simulink model "MPC_control"  (R2018a)
settings: Solver=FixedStepAuto  StartTime=0  StopTime=Tend  FixedStep=0.001  RelTol=5e-3
model workspace (MAT data in the model file):
  A_mu = 10
  B_reff = 8.386
  Cz = 7766.25
  DCT_Param : struct (value not decoded)
  D_reff = 0.25826
  Downshift_Speeds = [9.5625 12.9375 16.3125 19.6875 23.0625 26.4375 29.8125 33.1875 36.5625 39.9375 43.3125 46.6875 ... (28 elements, 4x7)]
  Pedal_Positions = [0.1 0.4 0.5 0.9]
  SUS : struct (value not decoded)
  Upshift_Speeds = [12.9375 16.3125 19.6875 33 26.4375 29.8125 33.1875 52.5 39.9375 43.3125 46.6875 77.25 ... (28 elements, 4x7)]
  VEH : struct (value not decoded)
  V_o = 16.7
  V_xlow = 1
  WH : struct (value not decoded)
  a = 1.4
  alpha_max = 1.5
  alpha_min = -1.5
  b = 1.8
  c_zo = 209651
  epsilon = 0.1
  h = 0.134
  path : struct (value not decoded)
  pio = 220000
  q_Fcx = 0
  q_Fz2 = 15.4
  q_Fzy = 0
  q_reo = 0.9974
  q_sx1 = -0.007764
  q_sx10 = 0.2824
  q_sx11 = 5.349
  q_sx12 = 0
  q_sx13 = 0
  q_sx14 = 0
  q_sx2 = 1.1915
  q_sx3 = 0.013948
  q_sx4 = 4.912
  q_sx5 = 1.02
  q_sx6 = 22.83
  q_sx7 = 0.7104
  q_sx8 = -0.023393
  q_sx9 = 0.6581
  q_sy1 = 0.00702
  q_sy2 = 0
  q_sy3 = 0.001515
  q_sy4 = 8.514e-05
  q_sy5 = 0
  q_sy6 = 0
  q_sy7 = 0.9008
  q_sy8 = -0.4089
  q_v1 = 0.0007742
  q_v2 = 0.04667
  r_Bx1 = 12.531
  r_Bx2 = 9.532
  r_Bx3 = 0
  r_By1 = 10.615
  r_By2 = 7.705
  r_By3 = 3.433e-06
  r_By4 = 0
  r_Cx1 = 1.019
  r_Cy1 = 1.0585
  r_Ex1 = -0.4487
  r_Ex2 = -0.4726
  r_Ey1 = 0.3132
  r_Ey2 = 7.63e-06
  r_Hx1 = 0.0002374
  r_Hy1 = 0.011646
  r_Hy2 = 7.63e-06
  r_Vy1 = 0.05654
  r_Vy2 = 7.63e-06
  r_Vy3 = 0
  r_Vy4 = 99.9
  r_Vy5 = 2
  r_Vy6 = 15.814
  r_o = 0.3135
  vehWidth = 2
  w = 1
symbols that are objects in the model workspace (value not decoded): VEH
undefined symbols (not defined in the file): Cok_1, Cok_2, Cok_3, Cok_4, Cok_5, Cok_6, Cok_7, Cok_8, Cok_9, Cout_1, Cout_2, Cout_3, Cout_4, Cout_5, Cout_6, Cout_7, Cout_8, Cout_9, DiscIntNeverNeededParam, Dout_1, Dout_2, Dout_3, Dout_4, Dout_5, Dout_6, Dout_7, Dout_8, Dout_9, F_1, F_2, F_3, F_4, F_5, F_6, F_7, F_8, F_9, Gd_1, Gd_2, Gd_3, Gd_4, Gd_5, Gd_6, Gd_7, Gd_8, Gd_9, Gok_1, Gok_2, Gok_3, Gok_4, Gok_5, Gok_6, Gok_7, Gok_8, Gok_9, Gsys_2, Gsys_9, Hd_1, Hd_2, Hd_3 ... (+70)
libraries: robotalgslib x10, simulink x5, sim3dlib x2, autolibutils x1, vehdynlibviscommon x1
(part 4 of 5)

== system MPC_control/observer_of_plant/Subsystem_3/simulator_3/VH2P ==
  Velocities : Inport
  HeadingAngles : Inport  Port=2
  Initial position : Inport  Port=3
  Iintial Velocities : Inport  Port=4
  Iintial HeadingAngles : Inport  Port=5
  select_overlap : Inport  Port=6
  From Workspace1 : FromWorkspace  VariableName=Tsim  SampleTime=Ts
  Resettable Delay1 : Delay  DelayLength=1  InitialConditionSource=Input port  ExternalReset=Rising  SampleTime=Ts
      settings: InputPortMap=u0,r5,p4
  Resettable Delay2 : Delay  DelayLength=1  InitialConditionSource=Input port  ExternalReset=Rising  SampleTime=Ts
      settings: InputPortMap=u0,r5,p4
  Resettable Delay3 : Delay  DelayLength=1  InitialConditionSource=Input port  ExternalReset=Rising  SampleTime=Ts
      settings: InputPortMap=u0,r5,p4
  To Workspace : ToWorkspace  VariableName=Heading3  SampleTime=-1
  To Workspace1 : ToWorkspace  VariableName=Velocity3  SampleTime=-1
  To Workspace2 : ToWorkspace  VariableName=LastVelocity3  SampleTime=-1
  To Workspace3 : ToWorkspace  VariableName=Lastposition3  SampleTime=-1
  To Workspace4 : ToWorkspace  VariableName=LastHeading3  SampleTime=-1
  Unit Delay2 : UnitDelay  SampleTime=Ts
  YV2P : MATLAB Function  TreatAsAtomicUnit=on  SystemSampleTime=Ts
  Position : Outport
  wires:
  Velocities/1 -> Resettable Delay1/1, To Workspace1/1, YV2P/1(Velocity)
  Resettable Delay1/1 -> YV2P/2(LastVelocity), To Workspace2/1
  HeadingAngles/1 -> Resettable Delay2/1, To Workspace/1, YV2P/3(Heading)
  Resettable Delay2/1 -> YV2P/4(LastHeading), To Workspace4/1
  Initial position/1 -> Resettable Delay3/3
  Iintial Velocities/1 -> Resettable Delay1/3
  Iintial HeadingAngles/1 -> Resettable Delay2/3
  select_overlap/1 -> Resettable Delay3/2, Resettable Delay2/2, Resettable Delay1/2
  From Workspace1/1 -> YV2P/5(Tsim), Unit Delay2/1
  Unit Delay2/1 -> YV2P/6(LastTsim)
  Resettable Delay3/1 -> YV2P/7(Lastpostion), To Workspace3/1
  YV2P/1(Position) -> Resettable Delay3/1, Position/1

== system MPC_control/observer_of_plant/Subsystem_3/simulator_3/YV_update ==
  XY_sim : Inport
  Velocity_sim : Inport  Port=2
  Heading_sim : Inport  Port=3
  Constant : Constant  Value=Ts  SampleTime=Ts
  Discrete-Time Integrator : DiscreteIntegrator  Commented=on  SampleTime=Ts  ICPrevOutput=DiscIntNeverNeededParam  ICPrevScaledInput=DiscIntNeverNeededParam
  From Workspace1 : FromWorkspace  VariableName=Tsim  SampleTime=Ts
  From Workspace3 : FromWorkspace  VariableName=XYplot_ref  SampleTime=Ts
  Gain : Gain  Commented=on  Gain=[eye(2), zeros(2,10)]  Multiplication=Matrix(K*u) (u vector)
  Mux : Mux  Commented=on  Inputs=2
  Pure Pursuit : robotalgslib/Pure Pursuit  Commented=on  DesiredLinearVelocity=0.1  MaxAngularVelocity=1.0  LookaheadDistance=2.5  TargetDirPort=off  SimulateUsing=Code generation
      settings: SourceProductName=Robotics System Toolbox  SourceProductBaseCode=RO
  Transpose : Math  Commented=on  Operator=transpose  SaturateOnIntegerOverflow=on
  YV_update : MATLAB Function  TreatAsAtomicUnit=on  SystemSampleTime=Ts
  Velocity_updated : Outport
  Heading_updated : Outport  Port=2
  wires:
  YV_update/1(Velocity_updated) -> Velocity_updated/1
  From Workspace1/1 -> YV_update/6(Tsim)
  Velocity_sim/1 -> YV_update/3(Velocity_sim)
  Constant/1 -> YV_update/5(Ts)
  Pure Pursuit/2 -> Discrete-Time Integrator/1
  Heading_sim/1 -> Mux/2, YV_update/4(Heading_sim)
  Mux/1 -> Pure Pursuit/1
  From Workspace3/1 -> Gain/1, YV_update/1(XYplot_ref)
  XY_sim/1 -> Mux/1, YV_update/2(XYplot_sim)
  Gain/1 -> Transpose/1
  Transpose/1 -> Pure Pursuit/2
  YV_update/2(Heading_updated) -> Heading_updated/1

== system MPC_control/observer_of_plant/Subsystem_4/simulator_4/MPC_of_simulator_4 ==
  Velocity_updated : Inport  SampleTime=Ts  LockScale=on
  Heading_updated : Inport  Port=2  SampleTime=Ts  LockScale=on
  Xhat : Inport  Port=3
  U(k-1) : Inport  Port=4  SampleTime=Ts  LockScale=on
  select_MPC : Inport  Port=5  SampleTime=Ts  LockScale=on
  select_overlap : Inport  Port=6  SampleTime=Ts  LockScale=on
  Clock : Clock
  Constant1 : Constant  Value=M  VectorParams1D=off  SampleTime=-1
  Constant2 : Constant  Value=Np  SampleTime=-1
  Constant3 : Constant  Value=JE_4  VectorParams1D=off  SampleTime=-1
  Constant4 : Constant  Value=Qc_4  VectorParams1D=off  SampleTime=-1
  Constant5 : Constant  Value=phi_4  VectorParams1D=off  SampleTime=-1
  F_Middle : Gain  Gain=F_4  Multiplication=Matrix(K*u) (u vector)
  From Workspace6 : FromWorkspace  VariableName=Rs  SampleTime=Ts
  HQP : MATLAB Function  TreatAsAtomicUnit=on  SystemSampleTime=Ts
  Resettable Delay2 : Delay  DelayLength=1  InitialConditionSource=Input port  ExternalReset=Rising  SampleTime=Ts
      settings: InputPortMap=u0,r5,p4
  r(k+1) : Outport
  U : Outport  Port=2
  wires:
  HQP/2(U) -> Resettable Delay2/1, U/1
  Xhat/1 -> F_Middle/1
  Constant4/1 -> HQP/4(Qc)
  Constant5/1 -> HQP/2(phi)
  Constant3/1 -> HQP/1(JE)
  Constant2/1 -> HQP/6(Np)
  Constant1/1 -> HQP/5(M)
  Clock/1 -> HQP/10(Tsim)
  F_Middle/1 -> HQP/3(Fxh)
  From Workspace6/1 -> HQP/9(Rs)
  Heading_updated/1 -> HQP/7(Heading_updated)
  Velocity_updated/1 -> HQP/8(Velocity_updated)
  HQP/1(r) -> r(k+1)/1
  select_MPC/1 -> HQP/11(select_MPC)
  Resettable Delay2/1 -> HQP/12(U_delay)
  select_overlap/1 -> HQP/13(select_overlap), Resettable Delay2/2
  U(k-1)/1 -> Resettable Delay2/3

== system MPC_control/observer_of_plant/Subsystem_4/simulator_4/VH2P ==
  Velocities : Inport
  HeadingAngles : Inport  Port=2
  Initial position : Inport  Port=3
  Iintial Velocities : Inport  Port=4
  Iintial HeadingAngles : Inport  Port=5
  select_overlap : Inport  Port=6
  From Workspace1 : FromWorkspace  VariableName=Tsim  SampleTime=Ts
  Resettable Delay1 : Delay  DelayLength=1  InitialConditionSource=Input port  ExternalReset=Rising  SampleTime=Ts
      settings: InputPortMap=u0,r5,p4
  Resettable Delay2 : Delay  DelayLength=1  InitialConditionSource=Input port  ExternalReset=Rising  SampleTime=Ts
      settings: InputPortMap=u0,r5,p4
  Resettable Delay3 : Delay  DelayLength=1  InitialConditionSource=Input port  ExternalReset=Rising  SampleTime=Ts
      settings: InputPortMap=u0,r5,p4
  Unit Delay2 : UnitDelay  SampleTime=Ts
  YV2P : MATLAB Function  TreatAsAtomicUnit=on  SystemSampleTime=Ts
  Position : Outport
  wires:
  YV2P/1(Position) -> Resettable Delay3/1, Position/1
  Velocities/1 -> Resettable Delay1/1, YV2P/1(Velocity)
  Resettable Delay1/1 -> YV2P/2(LastVelocity)
  HeadingAngles/1 -> Resettable Delay2/1, YV2P/3(Heading)
  Resettable Delay2/1 -> YV2P/4(LastHeading)
  Resettable Delay3/1 -> YV2P/7(Lastpostion)
  Initial position/1 -> Resettable Delay3/3
  Iintial Velocities/1 -> Resettable Delay1/3
  Iintial HeadingAngles/1 -> Resettable Delay2/3
  select_overlap/1 -> Resettable Delay3/2, Resettable Delay2/2, Resettable Delay1/2
  From Workspace1/1 -> YV2P/5(Tsim), Unit Delay2/1
  Unit Delay2/1 -> YV2P/6(LastTsim)

== system MPC_control/observer_of_plant/Subsystem_4/simulator_4/YV_update ==
  XY_sim : Inport
  Velocity_sim : Inport  Port=2
  Heading_sim : Inport  Port=3
  Constant : Constant  Value=Ts  SampleTime=Ts
  Discrete-Time Integrator : DiscreteIntegrator  Commented=on  SampleTime=Ts  ICPrevOutput=DiscIntNeverNeededParam  ICPrevScaledInput=DiscIntNeverNeededParam
  From Workspace1 : FromWorkspace  VariableName=Tsim  SampleTime=Ts
  From Workspace3 : FromWorkspace  VariableName=XYplot_ref  SampleTime=Ts
  Gain : Gain  Commented=on  Gain=[eye(2), zeros(2,10)]  Multiplication=Matrix(K*u) (u vector)
  Mux : Mux  Commented=on  Inputs=2
  Pure Pursuit : robotalgslib/Pure Pursuit  Commented=on  DesiredLinearVelocity=0.1  MaxAngularVelocity=1.0  LookaheadDistance=2.5  TargetDirPort=off  SimulateUsing=Code generation
      settings: SourceProductName=Robotics System Toolbox  SourceProductBaseCode=RO
  Transpose : Math  Commented=on  Operator=transpose  SaturateOnIntegerOverflow=on
  YV_update : MATLAB Function  TreatAsAtomicUnit=on  SystemSampleTime=Ts
  Velocity_updated : Outport
  Heading_updated : Outport  Port=2
  wires:
  From Workspace1/1 -> YV_update/6(Tsim)
  Velocity_sim/1 -> YV_update/3(Velocity_sim)
  Constant/1 -> YV_update/5(Ts)
  Pure Pursuit/2 -> Discrete-Time Integrator/1
  Heading_sim/1 -> Mux/2, YV_update/4(Heading_sim)
  From Workspace3/1 -> Gain/1, YV_update/1(XYplot_ref)
  Mux/1 -> Pure Pursuit/1
  YV_update/1(Velocity_updated) -> Velocity_updated/1
  Transpose/1 -> Pure Pursuit/2
  Gain/1 -> Transpose/1
  XY_sim/1 -> Mux/1, YV_update/2(XYplot_sim)
  YV_update/2(Heading_updated) -> Heading_updated/1

== system MPC_control/observer_of_plant/Subsystem_5/simulator_5/MPC_of_simulator_5 ==
  Velocity_updated : Inport  SampleTime=Ts  LockScale=on
  Heading_updated : Inport  Port=2  SampleTime=Ts  LockScale=on
  Xhat : Inport  Port=3
  U(k-1) : Inport  Port=4  SampleTime=Ts  LockScale=on
  select_MPC : Inport  Port=5  SampleTime=Ts  LockScale=on
  select_overlap : Inport  Port=6  SampleTime=Ts  LockScale=on
  Clock : Clock
  Constant1 : Constant  Value=M  VectorParams1D=off  SampleTime=-1
  Constant2 : Constant  Value=Np  SampleTime=-1
  Constant3 : Constant  Value=JE_5  VectorParams1D=off  SampleTime=-1
  Constant4 : Constant  Value=Qc_5  VectorParams1D=off  SampleTime=-1
  Constant5 : Constant  Value=phi_5  VectorParams1D=off  SampleTime=-1
  F_Middle : Gain  Gain=F_5  Multiplication=Matrix(K*u) (u vector)
  From Workspace6 : FromWorkspace  VariableName=Rs  SampleTime=Ts
  HQP : MATLAB Function  TreatAsAtomicUnit=on  SystemSampleTime=Ts
  Resettable Delay2 : Delay  DelayLength=1  InitialConditionSource=Input port  ExternalReset=Rising  SampleTime=Ts
      settings: InputPortMap=u0,r5,p4
  r(k+1) : Outport
  U : Outport  Port=2
  wires:
  HQP/2(U) -> Resettable Delay2/1, U/1
  Xhat/1 -> F_Middle/1
  Constant4/1 -> HQP/4(Qc)
  Constant5/1 -> HQP/2(phi)
  Constant3/1 -> HQP/1(JE)
  Constant2/1 -> HQP/6(Np)
  Constant1/1 -> HQP/5(M)
  Clock/1 -> HQP/10(Tsim)
  F_Middle/1 -> HQP/3(Fxh)
  From Workspace6/1 -> HQP/9(Rs)
  Heading_updated/1 -> HQP/7(Heading_updated)
  Velocity_updated/1 -> HQP/8(Velocity_updated)
  HQP/1(r) -> r(k+1)/1
  select_MPC/1 -> HQP/11(select_MPC)
  Resettable Delay2/1 -> HQP/12(U_delay)
  select_overlap/1 -> Resettable Delay2/2
  U(k-1)/1 -> Resettable Delay2/3

== system MPC_control/observer_of_plant/Subsystem_5/simulator_5/VH2P ==
  Velocities : Inport
  HeadingAngles : Inport  Port=2
  Initial position : Inport  Port=3
  Iintial Velocities : Inport  Port=4
  Iintial HeadingAngles : Inport  Port=5
  select_overlap : Inport  Port=6
  From Workspace1 : FromWorkspace  VariableName=Tsim  SampleTime=Ts
  Resettable Delay1 : Delay  DelayLength=1  InitialConditionSource=Input port  ExternalReset=Rising  SampleTime=Ts
      settings: InputPortMap=u0,r5,p4
  Resettable Delay2 : Delay  DelayLength=1  InitialConditionSource=Input port  ExternalReset=Rising  SampleTime=Ts
      settings: InputPortMap=u0,r5,p4
  Resettable Delay3 : Delay  DelayLength=1  InitialConditionSource=Input port  ExternalReset=Rising  SampleTime=Ts
      settings: InputPortMap=u0,r5,p4
  Unit Delay2 : UnitDelay  SampleTime=Ts
  YV2P : MATLAB Function  TreatAsAtomicUnit=on  SystemSampleTime=Ts
  Position : Outport
  wires:
  YV2P/1(Position) -> Resettable Delay3/1, Position/1
  Velocities/1 -> Resettable Delay1/1, YV2P/1(Velocity)
  Resettable Delay1/1 -> YV2P/2(LastVelocity)
  HeadingAngles/1 -> Resettable Delay2/1, YV2P/3(Heading)
  Resettable Delay2/1 -> YV2P/4(LastHeading)
  Resettable Delay3/1 -> YV2P/7(Lastpostion)
  Initial position/1 -> Resettable Delay3/3
  Iintial Velocities/1 -> Resettable Delay1/3
  Iintial HeadingAngles/1 -> Resettable Delay2/3
  select_overlap/1 -> Resettable Delay3/2, Resettable Delay2/2, Resettable Delay1/2
  From Workspace1/1 -> YV2P/5(Tsim), Unit Delay2/1
  Unit Delay2/1 -> YV2P/6(LastTsim)

== system MPC_control/observer_of_plant/Subsystem_5/simulator_5/YV_update ==
  XY_sim : Inport
  Velocity_sim : Inport  Port=2
  Heading_sim : Inport  Port=3
  Constant : Constant  Value=Ts  SampleTime=Ts
  Discrete-Time Integrator : DiscreteIntegrator  Commented=on  SampleTime=Ts  ICPrevOutput=DiscIntNeverNeededParam  ICPrevScaledInput=DiscIntNeverNeededParam
  From Workspace1 : FromWorkspace  VariableName=Tsim  SampleTime=Ts
  From Workspace3 : FromWorkspace  VariableName=XYplot_ref  SampleTime=Ts
  Gain : Gain  Commented=on  Gain=[eye(2), zeros(2,10)]  Multiplication=Matrix(K*u) (u vector)
  Mux : Mux  Commented=on  Inputs=2
  Pure Pursuit : robotalgslib/Pure Pursuit  Commented=on  DesiredLinearVelocity=0.1  MaxAngularVelocity=1.0  LookaheadDistance=2.5  TargetDirPort=off  SimulateUsing=Code generation
      settings: SourceProductName=Robotics System Toolbox  SourceProductBaseCode=RO
  Transpose : Math  Commented=on  Operator=transpose  SaturateOnIntegerOverflow=on
  YV_update : MATLAB Function  TreatAsAtomicUnit=on  SystemSampleTime=Ts
  Velocity_updated : Outport
  Heading_updated : Outport  Port=2
  wires:
  YV_update/1(Velocity_updated) -> Velocity_updated/1
  From Workspace1/1 -> YV_update/6(Tsim)
  Velocity_sim/1 -> YV_update/3(Velocity_sim)
  Constant/1 -> YV_update/5(Ts)
  Pure Pursuit/2 -> Discrete-Time Integrator/1
  Heading_sim/1 -> Mux/2, YV_update/4(Heading_sim)
  Mux/1 -> Pure Pursuit/1
  From Workspace3/1 -> Gain/1, YV_update/1(XYplot_ref)
  XY_sim/1 -> Mux/1, YV_update/2(XYplot_sim)
  Gain/1 -> Transpose/1
  Transpose/1 -> Pure Pursuit/2
  YV_update/2(Heading_updated) -> Heading_updated/1

== system MPC_control/observer_of_plant/Subsystem_6/simulator_6/MPC_of_simulator_6 ==
  Velocity_updated : Inport  SampleTime=Ts  LockScale=on
  Heading_updated : Inport  Port=2  SampleTime=Ts  LockScale=on
  Xhat : Inport  Port=3
  U(k-1) : Inport  Port=4  SampleTime=Ts  LockScale=on
  select_MPC : Inport  Port=5  SampleTime=Ts  LockScale=on
  select_overlap : Inport  Port=6  SampleTime=Ts  LockScale=on
  Clock : Clock
  Constant1 : Constant  Value=M  VectorParams1D=off  SampleTime=-1
  Constant2 : Constant  Value=Np  SampleTime=-1
  Constant3 : Constant  Value=JE_6  VectorParams1D=off  SampleTime=-1
  Constant4 : Constant  Value=Qc_6  VectorParams1D=off  SampleTime=-1
  Constant5 : Constant  Value=phi_6  VectorParams1D=off  SampleTime=-1
  F_Middle : Gain  Gain=F_6  Multiplication=Matrix(K*u) (u vector)
  From Workspace6 : FromWorkspace  VariableName=Rs  SampleTime=Ts
  HQP : MATLAB Function  TreatAsAtomicUnit=on  SystemSampleTime=Ts
  Resettable Delay2 : Delay  DelayLength=1  InitialConditionSource=Input port  ExternalReset=Rising  SampleTime=Ts
      settings: InputPortMap=u0,r5,p4
  r(k+1) : Outport
  U : Outport  Port=2
  wires:
  HQP/2(U) -> Resettable Delay2/1, U/1
  Xhat/1 -> F_Middle/1
  Constant4/1 -> HQP/4(Qc)
  Constant5/1 -> HQP/2(phi)
  Constant3/1 -> HQP/1(JE)
  Constant2/1 -> HQP/6(Np)
  Constant1/1 -> HQP/5(M)
  Clock/1 -> HQP/10(Tsim)
  F_Middle/1 -> HQP/3(Fxh)
  From Workspace6/1 -> HQP/9(Rs)
  Heading_updated/1 -> HQP/7(Heading_updated)
  Velocity_updated/1 -> HQP/8(Velocity_updated)
  HQP/1(r) -> r(k+1)/1
  select_MPC/1 -> HQP/11(select_MPC)
  Resettable Delay2/1 -> HQP/12(U_delay)
  select_overlap/1 -> Resettable Delay2/2
  U(k-1)/1 -> Resettable Delay2/3

== system MPC_control/observer_of_plant/Subsystem_6/simulator_6/VH2P ==
  Velocities : Inport
  HeadingAngles : Inport  Port=2
  Initial position : Inport  Port=3
  Iintial Velocities : Inport  Port=4
  Iintial HeadingAngles : Inport  Port=5
  select_overlap : Inport  Port=6
  From Workspace1 : FromWorkspace  VariableName=Tsim  SampleTime=Ts
  Resettable Delay1 : Delay  DelayLength=1  InitialConditionSource=Input port  ExternalReset=Rising  SampleTime=Ts
      settings: InputPortMap=u0,r5,p4
  Resettable Delay2 : Delay  DelayLength=1  InitialConditionSource=Input port  ExternalReset=Rising  SampleTime=Ts
      settings: InputPortMap=u0,r5,p4
  Resettable Delay3 : Delay  DelayLength=1  InitialConditionSource=Input port  ExternalReset=Rising  SampleTime=Ts
      settings: InputPortMap=u0,r5,p4
  Unit Delay2 : UnitDelay  SampleTime=Ts
  YV2P : MATLAB Function  TreatAsAtomicUnit=on  SystemSampleTime=Ts
  Position : Outport
  wires:
  YV2P/1(Position) -> Resettable Delay3/1, Position/1
  Velocities/1 -> Resettable Delay1/1, YV2P/1(Velocity)
  Resettable Delay1/1 -> YV2P/2(LastVelocity)
  HeadingAngles/1 -> Resettable Delay2/1, YV2P/3(Heading)
  Resettable Delay2/1 -> YV2P/4(LastHeading)
  Resettable Delay3/1 -> YV2P/7(Lastpostion)
  Initial position/1 -> Resettable Delay3/3
  Iintial Velocities/1 -> Resettable Delay1/3
  Iintial HeadingAngles/1 -> Resettable Delay2/3
  select_overlap/1 -> Resettable Delay3/2, Resettable Delay2/2, Resettable Delay1/2
  From Workspace1/1 -> YV2P/5(Tsim), Unit Delay2/1
  Unit Delay2/1 -> YV2P/6(LastTsim)

== system MPC_control/observer_of_plant/Subsystem_6/simulator_6/YV_update ==
  XY_sim : Inport
  Velocity_sim : Inport  Port=2
  Heading_sim : Inport  Port=3
  Constant : Constant  Value=Ts  SampleTime=Ts
  Discrete-Time Integrator : DiscreteIntegrator  Commented=on  SampleTime=Ts  ICPrevOutput=DiscIntNeverNeededParam  ICPrevScaledInput=DiscIntNeverNeededParam
  From Workspace1 : FromWorkspace  VariableName=Tsim  SampleTime=Ts
  From Workspace3 : FromWorkspace  VariableName=XYplot_ref  SampleTime=Ts
  Gain : Gain  Commented=on  Gain=[eye(2), zeros(2,10)]  Multiplication=Matrix(K*u) (u vector)
  Mux : Mux  Commented=on  Inputs=2
  Pure Pursuit : robotalgslib/Pure Pursuit  Commented=on  DesiredLinearVelocity=0.1  MaxAngularVelocity=1.0  LookaheadDistance=2.5  TargetDirPort=off  SimulateUsing=Code generation
      settings: SourceProductName=Robotics System Toolbox  SourceProductBaseCode=RO
  Transpose : Math  Commented=on  Operator=transpose  SaturateOnIntegerOverflow=on
  YV_update : MATLAB Function  TreatAsAtomicUnit=on  SystemSampleTime=Ts
  Velocity_updated : Outport
  Heading_updated : Outport  Port=2
  wires:
  YV_update/1(Velocity_updated) -> Velocity_updated/1
  From Workspace1/1 -> YV_update/6(Tsim)
  Velocity_sim/1 -> YV_update/3(Velocity_sim)
  Constant/1 -> YV_update/5(Ts)
  Pure Pursuit/2 -> Discrete-Time Integrator/1
  Heading_sim/1 -> Mux/2, YV_update/4(Heading_sim)
  Mux/1 -> Pure Pursuit/1
  From Workspace3/1 -> Gain/1, YV_update/1(XYplot_ref)
  XY_sim/1 -> Mux/1, YV_update/2(XYplot_sim)
  Gain/1 -> Transpose/1
  Transpose/1 -> Pure Pursuit/2
  YV_update/2(Heading_updated) -> Heading_updated/1

== system MPC_control/observer_of_plant/Subsystem_7/simulator_7/MPC_of_simulator_7 ==
  Velocity_updated : Inport  SampleTime=Ts  LockScale=on
  Heading_updated : Inport  Port=2  SampleTime=Ts  LockScale=on
  Xhat : Inport  Port=3
  U(k-1) : Inport  Port=4  SampleTime=Ts  LockScale=on
  select_MPC : Inport  Port=5  SampleTime=Ts  LockScale=on
  select_overlap : Inport  Port=6  SampleTime=Ts  LockScale=on
  Clock : Clock
  Constant1 : Constant  Value=M  VectorParams1D=off  SampleTime=-1
  Constant2 : Constant  Value=Np  SampleTime=-1
  Constant3 : Constant  Value=JE_7  VectorParams1D=off  SampleTime=-1
  Constant4 : Constant  Value=Qc_7  VectorParams1D=off  SampleTime=-1
  Constant5 : Constant  Value=phi_7  VectorParams1D=off  SampleTime=-1
  F_Middle : Gain  Gain=F_7  Multiplication=Matrix(K*u) (u vector)
  From Workspace6 : FromWorkspace  VariableName=Rs  SampleTime=Ts
  HQP : MATLAB Function  TreatAsAtomicUnit=on  SystemSampleTime=Ts
  Resettable Delay2 : Delay  DelayLength=1  InitialConditionSource=Input port  ExternalReset=Rising  SampleTime=Ts
      settings: InputPortMap=u0,r5,p4
  r(k+1) : Outport
  U : Outport  Port=2
  wires:
  HQP/2(U) -> Resettable Delay2/1, U/1
  Xhat/1 -> F_Middle/1
  Constant4/1 -> HQP/4(Qc)
  Constant5/1 -> HQP/2(phi)
  Constant3/1 -> HQP/1(JE)
  Constant2/1 -> HQP/6(Np)
  Constant1/1 -> HQP/5(M)
  Clock/1 -> HQP/10(Tsim)
  F_Middle/1 -> HQP/3(Fxh)
  From Workspace6/1 -> HQP/9(Rs)
  Heading_updated/1 -> HQP/7(Heading_updated)
  Velocity_updated/1 -> HQP/8(Velocity_updated)
  HQP/1(r) -> r(k+1)/1
  select_MPC/1 -> HQP/11(select_MPC)
  Resettable Delay2/1 -> HQP/12(U_delay)
  select_overlap/1 -> Resettable Delay2/2
  U(k-1)/1 -> Resettable Delay2/3

== system MPC_control/observer_of_plant/Subsystem_7/simulator_7/VH2P ==
  Velocities : Inport
  HeadingAngles : Inport  Port=2
  Initial position : Inport  Port=3
  Iintial Velocities : Inport  Port=4
  Iintial HeadingAngles : Inport  Port=5
  select_overlap : Inport  Port=6
  From Workspace1 : FromWorkspace  VariableName=Tsim  SampleTime=Ts
  Resettable Delay1 : Delay  DelayLength=1  InitialConditionSource=Input port  ExternalReset=Rising  SampleTime=Ts
      settings: InputPortMap=u0,r5,p4
  Resettable Delay2 : Delay  DelayLength=1  InitialConditionSource=Input port  ExternalReset=Rising  SampleTime=Ts
      settings: InputPortMap=u0,r5,p4
  Resettable Delay3 : Delay  DelayLength=1  InitialConditionSource=Input port  ExternalReset=Rising  SampleTime=Ts
      settings: InputPortMap=u0,r5,p4
  Unit Delay2 : UnitDelay  SampleTime=Ts
  YV2P : MATLAB Function  TreatAsAtomicUnit=on  SystemSampleTime=Ts
  Position : Outport
  wires:
  YV2P/1(Position) -> Resettable Delay3/1, Position/1
  Resettable Delay2/1 -> YV2P/4(LastHeading)
  Resettable Delay3/1 -> YV2P/7(Lastpostion)
  Initial position/1 -> Resettable Delay3/3
  Iintial Velocities/1 -> Resettable Delay1/3
  Iintial HeadingAngles/1 -> Resettable Delay2/3
  select_overlap/1 -> Resettable Delay3/2, Resettable Delay2/2, Resettable Delay1/2
  From Workspace1/1 -> YV2P/5(Tsim), Unit Delay2/1
  Unit Delay2/1 -> YV2P/6(LastTsim)
  Resettable Delay1/1 -> YV2P/2(LastVelocity)
  HeadingAngles/1 -> Resettable Delay2/1, YV2P/3(Heading)
  Velocities/1 -> Resettable Delay1/1, YV2P/1(Velocity)

== system MPC_control/observer_of_plant/Subsystem_7/simulator_7/YV_update ==
  XY_sim : Inport
  Velocity_sim : Inport  Port=2
  Heading_sim : Inport  Port=3
  Constant : Constant  Value=Ts  SampleTime=Ts
  Discrete-Time Integrator : DiscreteIntegrator  Commented=on  SampleTime=Ts  ICPrevOutput=DiscIntNeverNeededParam  ICPrevScaledInput=DiscIntNeverNeededParam
  From Workspace1 : FromWorkspace  VariableName=Tsim  SampleTime=Ts
  From Workspace3 : FromWorkspace  VariableName=XYplot_ref  SampleTime=Ts
  Gain : Gain  Commented=on  Gain=[eye(2), zeros(2,10)]  Multiplication=Matrix(K*u) (u vector)
  Mux : Mux  Commented=on  Inputs=2
  Pure Pursuit : robotalgslib/Pure Pursuit  Commented=on  DesiredLinearVelocity=0.1  MaxAngularVelocity=1.0  LookaheadDistance=2.5  TargetDirPort=off  SimulateUsing=Code generation
      settings: SourceProductName=Robotics System Toolbox  SourceProductBaseCode=RO
  Transpose : Math  Commented=on  Operator=transpose  SaturateOnIntegerOverflow=on
  YV_update : MATLAB Function  TreatAsAtomicUnit=on  SystemSampleTime=Ts
  Velocity_updated : Outport
  Heading_updated : Outport  Port=2
  wires:
  From Workspace1/1 -> YV_update/6(Tsim)
  Velocity_sim/1 -> YV_update/3(Velocity_sim)
  Constant/1 -> YV_update/5(Ts)
  Pure Pursuit/2 -> Discrete-Time Integrator/1
  Heading_sim/1 -> Mux/2, YV_update/4(Heading_sim)
  From Workspace3/1 -> Gain/1, YV_update/1(XYplot_ref)
  YV_update/1(Velocity_updated) -> Velocity_updated/1
  Mux/1 -> Pure Pursuit/1
  Transpose/1 -> Pure Pursuit/2
  Gain/1 -> Transpose/1
  XY_sim/1 -> Mux/1, YV_update/2(XYplot_sim)
  YV_update/2(Heading_updated) -> Heading_updated/1

== system MPC_control/observer_of_plant/Subsystem_8/simulator_8/MPC_of_simulator_8 ==
  Velocity_updated : Inport  SampleTime=Ts  LockScale=on
  Heading_updated : Inport  Port=2  SampleTime=Ts  LockScale=on
  Xhat : Inport  Port=3
  U(k-1) : Inport  Port=4  SampleTime=Ts  LockScale=on
  select_MPC : Inport  Port=5  SampleTime=Ts  LockScale=on
  select_overlap : Inport  Port=6  SampleTime=Ts  LockScale=on
  Clock : Clock
  Constant1 : Constant  Value=M  VectorParams1D=off  SampleTime=-1
  Constant2 : Constant  Value=Np  SampleTime=-1
  Constant3 : Constant  Value=JE_8  VectorParams1D=off  SampleTime=-1
  Constant4 : Constant  Value=Qc_8  VectorParams1D=off  SampleTime=-1
  Constant5 : Constant  Value=phi_8  VectorParams1D=off  SampleTime=-1
  F_Middle1 : Gain  Gain=F_8  Multiplication=Matrix(K*u) (u vector)
  From Workspace6 : FromWorkspace  VariableName=Rs  SampleTime=Ts
  HQP : MATLAB Function  TreatAsAtomicUnit=on  SystemSampleTime=Ts
  Resettable Delay2 : Delay  DelayLength=1  InitialConditionSource=Input port  ExternalReset=Rising  SampleTime=Ts
      settings: InputPortMap=u0,r5,p4
  r(k+1) : Outport
  U : Outport  Port=2
  wires:
  HQP/2(U) -> Resettable Delay2/1, U/1
  Constant4/1 -> HQP/4(Qc)
  Constant5/1 -> HQP/2(phi)
  Constant3/1 -> HQP/1(JE)
  Constant2/1 -> HQP/6(Np)
  Constant1/1 -> HQP/5(M)
  Clock/1 -> HQP/10(Tsim)
  F_Middle1/1 -> HQP/3(Fxh)
  From Workspace6/1 -> HQP/9(Rs)
  Heading_updated/1 -> HQP/7(Heading_updated)
  Velocity_updated/1 -> HQP/8(Velocity_updated)
  HQP/1(r) -> r(k+1)/1
  select_MPC/1 -> HQP/11(select_MPC)
  Resettable Delay2/1 -> HQP/12(U_delay)
  select_overlap/1 -> Resettable Delay2/2
  U(k-1)/1 -> Resettable Delay2/3
  Xhat/1 -> F_Middle1/1

== system MPC_control/observer_of_plant/Subsystem_8/simulator_8/VH2P ==
  Velocities : Inport
  HeadingAngles : Inport  Port=2
  Initial position : Inport  Port=3
  Iintial Velocities : Inport  Port=4
  Iintial HeadingAngles : Inport  Port=5
  select_overlap : Inport  Port=6
  From Workspace1 : FromWorkspace  VariableName=Tsim  SampleTime=Ts
  Resettable Delay1 : Delay  DelayLength=1  InitialConditionSource=Input port  ExternalReset=Rising  SampleTime=Ts
      settings: InputPortMap=u0,r5,p4
  Resettable Delay2 : Delay  DelayLength=1  InitialConditionSource=Input port  ExternalReset=Rising  SampleTime=Ts
      settings: InputPortMap=u0,r5,p4
  Resettable Delay3 : Delay  DelayLength=1  InitialConditionSource=Input port  ExternalReset=Rising  SampleTime=Ts
      settings: InputPortMap=u0,r5,p4
  To Workspace : ToWorkspace  VariableName=Heading8  SampleTime=-1
  To Workspace1 : ToWorkspace  VariableName=Velocity8  SampleTime=-1
  To Workspace2 : ToWorkspace  VariableName=LastVelocity8  SampleTime=-1
  To Workspace3 : ToWorkspace  VariableName=Lastposition8  SampleTime=-1
  To Workspace4 : ToWorkspace  VariableName=LastHeading8  SampleTime=-1
  Unit Delay2 : UnitDelay  SampleTime=Ts
  YV2P : MATLAB Function  TreatAsAtomicUnit=on  SystemSampleTime=Ts
  Position : Outport
  wires:
  YV2P/1(Position) -> Resettable Delay3/1, Position/1
  Velocities/1 -> Resettable Delay1/1, To Workspace1/1, YV2P/1(Velocity)
  Resettable Delay1/1 -> To Workspace2/1, YV2P/2(LastVelocity)
  HeadingAngles/1 -> Resettable Delay2/1, To Workspace/1, YV2P/3(Heading)
  Resettable Delay2/1 -> To Workspace4/1, YV2P/4(LastHeading)
  Resettable Delay3/1 -> To Workspace3/1, YV2P/7(Lastpostion)
  Initial position/1 -> Resettable Delay3/3
  Iintial Velocities/1 -> Resettable Delay1/3
  Iintial HeadingAngles/1 -> Resettable Delay2/3
  select_overlap/1 -> Resettable Delay3/2, Resettable Delay2/2, Resettable Delay1/2
  From Workspace1/1 -> YV2P/5(Tsim), Unit Delay2/1
  Unit Delay2/1 -> YV2P/6(LastTsim)

== system MPC_control/observer_of_plant/Subsystem_8/simulator_8/YV_update ==
  XY_sim : Inport
  Velocity_sim : Inport  Port=2
  Heading_sim : Inport  Port=3
  Constant : Constant  Value=Ts  SampleTime=Ts
  Discrete-Time Integrator : DiscreteIntegrator  Commented=on  SampleTime=Ts  ICPrevOutput=DiscIntNeverNeededParam  ICPrevScaledInput=DiscIntNeverNeededParam
  From Workspace1 : FromWorkspace  VariableName=Tsim  SampleTime=Ts
  From Workspace3 : FromWorkspace  VariableName=XYplot_ref  SampleTime=Ts
  Gain : Gain  Commented=on  Gain=[eye(2), zeros(2,10)]  Multiplication=Matrix(K*u) (u vector)
  Mux : Mux  Commented=on  Inputs=2
  Pure Pursuit : robotalgslib/Pure Pursuit  Commented=on  DesiredLinearVelocity=0.1  MaxAngularVelocity=1.0  LookaheadDistance=2.5  TargetDirPort=off  SimulateUsing=Code generation
      settings: SourceProductName=Robotics System Toolbox  SourceProductBaseCode=RO
  Transpose : Math  Commented=on  Operator=transpose  SaturateOnIntegerOverflow=on
  YV_update : MATLAB Function  TreatAsAtomicUnit=on  SystemSampleTime=Ts
  Velocity_updated : Outport
  Heading_updated : Outport  Port=2
  wires:
  YV_update/1(Velocity_updated) -> Velocity_updated/1
  From Workspace1/1 -> YV_update/6(Tsim)
  Velocity_sim/1 -> YV_update/3(Velocity_sim)
  Constant/1 -> YV_update/5(Ts)
  Pure Pursuit/2 -> Discrete-Time Integrator/1
  Heading_sim/1 -> Mux/2, YV_update/4(Heading_sim)
  Mux/1 -> Pure Pursuit/1
  From Workspace3/1 -> YV_update/1(XYplot_ref), Gain/1
  XY_sim/1 -> Mux/1, YV_update/2(XYplot_sim)
  Gain/1 -> Transpose/1
  Transpose/1 -> Pure Pursuit/2
  YV_update/2(Heading_updated) -> Heading_updated/1

== system MPC_control/observer_of_plant/Subsystem_9/simulator_9/MPC_of_simulator_9 ==
  Velocity_updated : Inport  SampleTime=Ts  LockScale=on
  Heading_updated : Inport  Port=2  SampleTime=Ts  LockScale=on
  Xhat : Inport  Port=3
  U(k-1) : Inport  Port=4  SampleTime=Ts  LockScale=on
  select_MPC : Inport  Port=5  SampleTime=Ts  LockScale=on
  select_overlap : Inport  Port=6  SampleTime=Ts  LockScale=on
  Clock : Clock
  Constant1 : Constant  Value=M  VectorParams1D=off  SampleTime=-1
  Constant2 : Constant  Value=Np  SampleTime=-1
  Constant3 : Constant  Value=JE_9  VectorParams1D=off  SampleTime=-1
  Constant4 : Constant  Value=Qc_9  VectorParams1D=off  SampleTime=-1
  Constant5 : Constant  Value=phi_9  VectorParams1D=off  SampleTime=-1
  F_Middle : Gain  Gain=F_9  Multiplication=Matrix(K*u) (u vector)
  From Workspace6 : FromWorkspace  VariableName=Rs  SampleTime=Ts
  HQP : MATLAB Function  TreatAsAtomicUnit=on  SystemSampleTime=Ts
  Resettable Delay2 : Delay  DelayLength=1  InitialConditionSource=Input port  ExternalReset=Rising  SampleTime=Ts
      settings: InputPortMap=u0,r5,p4
  r(k+1) : Outport
  U : Outport  Port=2
  wires:
  HQP/2(U) -> Resettable Delay2/1, U/1
  Xhat/1 -> F_Middle/1
  Constant4/1 -> HQP/4(Qc)
  Constant5/1 -> HQP/2(phi)
  Constant3/1 -> HQP/1(JE)
  Constant2/1 -> HQP/6(Np)
  Constant1/1 -> HQP/5(M)
  Clock/1 -> HQP/10(Tsim)
  F_Middle/1 -> HQP/3(Fxh)
  From Workspace6/1 -> HQP/9(Rs)
  Heading_updated/1 -> HQP/7(Heading_updated)
  Velocity_updated/1 -> HQP/8(Velocity_updated)
  HQP/1(r) -> r(k+1)/1
  select_MPC/1 -> HQP/11(select_MPC)
  Resettable Delay2/1 -> HQP/12(U_delay)
  select_overlap/1 -> Resettable Delay2/2
  U(k-1)/1 -> Resettable Delay2/3

== system MPC_control/observer_of_plant/Subsystem_9/simulator_9/VH2P ==
  Velocities : Inport
  HeadingAngles : Inport  Port=2
  Initial position : Inport  Port=3
  Iintial Velocities : Inport  Port=4
  Iintial HeadingAngles : Inport  Port=5
  select_overlap : Inport  Port=6
  From Workspace1 : FromWorkspace  VariableName=Tsim  SampleTime=Ts
  Resettable Delay1 : Delay  DelayLength=1  InitialConditionSource=Input port  ExternalReset=Rising  SampleTime=Ts
      settings: InputPortMap=u0,r5,p4
  Resettable Delay2 : Delay  DelayLength=1  InitialConditionSource=Input port  ExternalReset=Rising  SampleTime=Ts
      settings: InputPortMap=u0,r5,p4
  Resettable Delay3 : Delay  DelayLength=1  InitialConditionSource=Input port  ExternalReset=Rising  SampleTime=Ts
      settings: InputPortMap=u0,r5,p4
  Unit Delay2 : UnitDelay  SampleTime=Ts
  YV2P : MATLAB Function  TreatAsAtomicUnit=on  SystemSampleTime=Ts
  Position : Outport
  wires:
  YV2P/1(Position) -> Resettable Delay3/1, Position/1
  Velocities/1 -> Resettable Delay1/1, YV2P/1(Velocity)
  Resettable Delay1/1 -> YV2P/2(LastVelocity)
  HeadingAngles/1 -> Resettable Delay2/1, YV2P/3(Heading)
  Resettable Delay2/1 -> YV2P/4(LastHeading)
  Resettable Delay3/1 -> YV2P/7(Lastpostion)
  Initial position/1 -> Resettable Delay3/3
  Iintial Velocities/1 -> Resettable Delay1/3
  Iintial HeadingAngles/1 -> Resettable Delay2/3
  select_overlap/1 -> Resettable Delay3/2, Resettable Delay2/2, Resettable Delay1/2
  From Workspace1/1 -> YV2P/5(Tsim), Unit Delay2/1
  Unit Delay2/1 -> YV2P/6(LastTsim)

== system MPC_control/observer_of_plant/Subsystem_9/simulator_9/YV_update ==
  XY_sim : Inport
  Velocity_sim : Inport  Port=2
  Heading_sim : Inport  Port=3
  Constant : Constant  Value=Ts  SampleTime=Ts
  Discrete-Time Integrator : DiscreteIntegrator  Commented=on  SampleTime=Ts  ICPrevOutput=DiscIntNeverNeededParam  ICPrevScaledInput=DiscIntNeverNeededParam
  From Workspace1 : FromWorkspace  VariableName=Tsim  SampleTime=Ts
  From Workspace3 : FromWorkspace  VariableName=XYplot_ref  SampleTime=Ts
  Gain : Gain  Commented=on  Gain=[eye(2), zeros(2,10)]  Multiplication=Matrix(K*u) (u vector)
  Mux : Mux  Commented=on  Inputs=2
  Pure Pursuit : robotalgslib/Pure Pursuit  Commented=on  DesiredLinearVelocity=0.1  MaxAngularVelocity=1.0  LookaheadDistance=2.5  TargetDirPort=off  SimulateUsing=Code generation
      settings: SourceProductName=Robotics System Toolbox  SourceProductBaseCode=RO
  Transpose : Math  Commented=on  Operator=transpose  SaturateOnIntegerOverflow=on
  YV_update : MATLAB Function  TreatAsAtomicUnit=on  SystemSampleTime=Ts
  Velocity_updated : Outport
  Heading_updated : Outport  Port=2
  wires:
  YV_update/1(Velocity_updated) -> Velocity_updated/1
  From Workspace1/1 -> YV_update/6(Tsim)
  Velocity_sim/1 -> YV_update/3(Velocity_sim)
  Constant/1 -> YV_update/5(Ts)
  Pure Pursuit/2 -> Discrete-Time Integrator/1
  Heading_sim/1 -> Mux/2, YV_update/4(Heading_sim)
  Mux/1 -> Pure Pursuit/1
  From Workspace3/1 -> Gain/1, YV_update/1(XYplot_ref)
  XY_sim/1 -> Mux/1, YV_update/2(XYplot_sim)
  Gain/1 -> Transpose/1
  Transpose/1 -> Pure Pursuit/2
  YV_update/2(Heading_updated) -> Heading_updated/1

== system MPC_control/Controllers/Brake Controller/Brake Pressure Control/Bang Bang ABS/Bang-bang controller ==
  in_1 : Inport
  Constant : Constant  Value=0
  Data Type Conversion1 : DataTypeConversion  OutDataTypeStr=double  SaturateOnIntegerOverflow=on  RndMeth=Zero
  Data Type Conversion2 : DataTypeConversion  OutDataTypeStr=double  SaturateOnIntegerOverflow=on  RndMeth=Zero
  Relational Operator : RelationalOperator  Operator=>  OutDataTypeStr=boolean  RndMeth=Nearest  InputSameDT=on
  Relational Operator1 : RelationalOperator  Operator=<  OutDataTypeStr=boolean  RndMeth=Nearest  InputSameDT=on
  Sum : Sum  Inputs=+-  SaturateOnIntegerOverflow=on  InputSameDT=on  OutDataTypeStr=Inherit: Same as first input
  out_1 : Outport  InitialOutput=0
  wires:
  Data Type Conversion2/1 -> Sum/2
  Data Type Conversion1/1 -> Sum/1
  Sum/1 -> out_1/1
  Relational Operator/1 -> Data Type Conversion1/1
  Relational Operator1/1 -> Data Type Conversion2/1
  Constant/1 -> Relational Operator/2, Relational Operator1/2
  in_1/1 -> Relational Operator1/1, Relational Operator/1

== system MPC_control/Visualization/3D Engine/3D Engine/Scale/PartConcatenation ==
  BodyX : Inport
  BodyY : Inport  Port=2
  BodyZ : Inport  Port=3
  WheelFrontLeftX : Inport  Port=4
  WheelFrontLeftY : Inport  Port=5
  WheelFrontLeftZ : Inport  Port=6
  WheelFrontRightX : Inport  Port=7
  WheelFrontRightY : Inport  Port=8
  WheelFrontRightZ : Inport  Port=9
  WheelRearLeftX : Inport  Port=10
  WheelRearLeftY : Inport  Port=11
  WheelRearLeftZ : Inport  Port=12
  WheelRearRightX : Inport  Port=13
  WheelRearRightY : Inport  Port=14
  WheelRearRightZ : Inport  Port=15
  AllParts : Concatenate  NumInputs=5  Mode=Multidimensional array
  Body : Concatenate  NumInputs=3  Mode=Multidimensional array  ConcatenateDimension=2
  WheelFrontLeft : Concatenate  NumInputs=3  Mode=Multidimensional array  ConcatenateDimension=2
  WheelFrontRight : Concatenate  NumInputs=3  Mode=Multidimensional array  ConcatenateDimension=2
  WheelRearLeft : Concatenate  NumInputs=3  Mode=Multidimensional array  ConcatenateDimension=2
  WheelRearRight : Concatenate  NumInputs=3  Mode=Multidimensional array  ConcatenateDimension=2
  ConcatOut : Outport
  wires:
  BodyX/1 -> Body/1
  BodyZ/1 -> Body/3
  WheelFrontLeftX/1 -> WheelFrontLeft/1
  WheelFrontLeftZ/1 -> WheelFrontLeft/3
  WheelFrontLeftY/1 -> WheelFrontLeft/2
  BodyY/1 -> Body/2
  WheelFrontLeft/1 -> AllParts/2
  WheelRearRightX/1 -> WheelRearRight/1
  Body/1 -> AllParts/1
  WheelRearLeft/1 -> AllParts/4
  WheelFrontRight/1 -> AllParts/3
  WheelRearRightZ/1 -> WheelRearRight/3
  WheelFrontRightY/1 -> WheelFrontRight/2
  WheelFrontRightX/1 -> WheelFrontRight/1
  WheelRearRightY/1 -> WheelRearRight/2
  WheelRearLeftZ/1 -> WheelRearLeft/3
  AllParts/1 -> ConcatOut/1
  WheelRearLeftY/1 -> WheelRearLeft/2
  WheelRearRight/1 -> AllParts/5
  WheelRearLeftX/1 -> WheelRearLeft/1
  WheelFrontRightZ/1 -> WheelFrontRight/3

== stateflow chart MPC_control/Controllers/Transmission Controller/TCM/TCM Shift Controller ==
  settings: sampleTime=0.01
  state GearState [parallel]
    settings: executionOrder=1
    state Neutral
      en:
      GearState = 0;
    state G1
      en:
      GearState = 1;
    state G2
      en:
      GearState = 2;
      du:
      [SpdThr] = calc(2,pedal,speed);
    state G3
      en:
      GearState = 3;
      du:
      [SpdThr] = calc(3,pedal,speed);
    state G8
      en:
      GearState = 8;
    state G7
      en:
      GearState = 7;
    state G6
      en:
      GearState = 6;
    state G5
      en:GearState=5;
      du:[SpdThr]=calc(5,pedal,speed);
    state G4
      en:
      GearState = 4;
      du:
      [SpdThr] = calc(4,pedal,speed);
    (default) -> G1
    Neutral -> G1 : [~Neutral]
    G1 -> G2 [order 1] : Up
    G2 -> G3 [order 1] : Up
    G1 -> Neutral [order 2] : [Neutral]
    G2 -> G1 [order 2] : Down
    G3 -> G2 [order 2] : Down
    G3 -> G4 [order 1] : Up
    G4 -> G3 [order 2] : Down
    G7 -> G8 [order 1] : Up
    G5 -> G6 [order 1] : Up
    G6 -> G7 [order 1] : Up
    G4 -> G5 [order 1] : Up
    G5 -> G4 [order 2] : Down
    G6 -> G5 [order 2] : Down
    G7 -> G6 [order 2] : Down
    G8 -> G7 : Down
  state SelectionState [parallel]
    du:[up_th]=calc_up(GearState,pedal);
    du:[down_th]=calc_down(GearState,pedal);
    settings: executionOrder=2
    state SteadyState
      en:
      clutchControl = 0;
    state preDownShifting
    state preUpShifting
    state UpShifting
      en:
      GearState = GearState + 0.5;
    state DownShifting
      en:
      GearState = GearState - 0.5;
    (default) -> SteadyState
    SteadyState -> (junction 62) [order 1] : [speed < down_th && ...
        | GearState >1]
    SteadyState -> (junction 128) [order 2] : [speed > up_th &&...
        | GearState <= 5 && ...
        | floor(GearState) == GearState]
    (junction 62) -> preDownShifting
    (junction 128) -> preUpShifting
    (junction 168) -> SteadyState
    (junction 23) -> SteadyState
    (junction 161) -> SteadyState
    preDownShifting -> (junction 168) [order 2] : [speed >= down_th]
    preUpShifting -> (junction 161) [order 2] : [speed <= up_th]
    preUpShifting -> UpShifting [order 1] : after(0.5,sec)
        | [speed>up_th]
    preDownShifting -> DownShifting [order 1] : after(0.5, sec)
        | [speed < down_th - 2]
    DownShifting -> (junction 23) : {GearState.Down;}
    UpShifting -> (junction 23) : {GearState.Up;}
  state up_th = calc_up(gear,pedal) [function]
  state down_th = calc_down(gear,pedal) [function]
  state SpdThr = calc(gear,pedal,speed) [function]
  data: gear function_input; pedal function_input; up_th function_output; gear function_input; pedal function_input; down_th function_output; gear function_input; pedal function_input; SpdThr function_output; speed function_input; GearState output int8; speed input; pedal input; clutchControl local double; SpdThr local double; Neutral input; up_th local double; down_th local double
  events: Up local EITHER_EDGE_EVENT; Down local EITHER_EDGE_EVENT

== matlab function MPC_control/Mpc_of_plant/HQP_solver ==
  data: select_MPC input; lambda output; r output; lamerr output; lamiter output; JE input; JF_part input; Fxh input; M input; Np input; U_min input; U_max input; Heading_updated input [1..5]; Velocity_updated input [1..5]; Rs input; Tsim input; Tend input; U_delay input; U output
function [lambda,r,lamerr,lamiter,U] = HQP_solver(select_MPC, JE, JF_part, Fxh, M, Np, U_min, U_max, Heading_updated, Velocity_updated, Rs, Tsim, Tend, U_delay)
U = zeros(2,1);
r = zeros(2,1);
lamerr = 0;
lamiter = 0;
[m,n] = size(M);
lambda = zeros(m,1);

du1_inc = 3*pi;du1_dec = 3*pi;
du2_inc = 1;du2_dec = 1;
dU_plus = []; dU_minus = [];
for i = 1:Np
    dU_plus = [dU_plus; [U_delay(1) + du1_inc; U_delay(2) + du2_inc]];
    dU_minus = [dU_minus; [-U_delay(1) + du1_dec; -U_delay(2) + du2_dec;]];
end
N = [U_max;
      U_min;
      dU_plus;
      dU_minus;          
     ];

if Tsim > 0 && select_MPC~=4 %&& select_MPC~=6 %&& select_MPC~=5 %&& select_MPC~=8
    for i = 1: Np  
        Rs(2*i-1,:) = Velocity_updated(i,:);
        Rs(2*i,:) = Heading_updated(i,:);
    end
end
% Rs(2,:) = Heading_updated;

JF = JF_part*(Rs-Fxh);
[u,lambda,lamerr,lamiter]= HQP(JE,JF,M,N);
U = u(1:2);
r = Rs(1:2,:);
end

== matlab function MPC_control/MATLAB Function ==
  data: u input; Tr output; Br output
function [Tr, Br] = choose(u)
Tr = 0; Br = 0;
if u > 0 || u == 0
    Tr = u;
else
    Br = abs(u);
end
end

== matlab function MPC_control/observer_of_plant/Subsystem_7/simulator_7/VH2P/YV2P ==
  data: Velocity input; LastVelocity input; Heading input; LastHeading input; Tsim input; LastTsim input; Lastpostion input; Position output
function Position  = YV2P(Velocity,LastVelocity, Heading, LastHeading, Tsim, LastTsim, Lastpostion)
if Tsim >= 0.1
    Position = zeros(2,1);
    X0 = Lastpostion(1,:); Y0 = Lastpostion(2,:);
    Vx0 = [LastVelocity*cos(LastHeading); Velocity*cos(Heading)];
    Vy0 = [LastVelocity*sin(LastHeading); Velocity*sin(Heading)];
    Yaw_sim = [LastHeading; Heading];
    T =[LastTsim; Tsim];
    [ X_tmp, Y_tmp] = YV2P( T, X0, Y0, Vx0, Vy0, Yaw_sim, zeros(2,1) );
    Position = [X_tmp(end,:); Y_tmp(end,:)];
else
    Position = [0; 0];
end
end

== matlab function MPC_control/observer_of_plant/Subsystem_7/simulator_7/YV_update/YV_update ==
  data: XYplot_ref input; Velocity_updated output; XYplot_sim input; Velocity_sim input; Heading_sim input; Ts input; Tsim input; Heading_updated output
function [Velocity_updated, Heading_updated] = VY_update(XYplot_ref, XYplot_sim, Velocity_sim, Heading_sim, Ts, Tsim)
Np = 6;
 disp(sprintf('Simulation time : %2.1f sec',Tsim)) 
 Heading_updated = zeros(Np,1); Velocity_updated = zeros(Np,1);
coder.extrinsic('P2YV');
T = []; 
for j = 1:Np+1
    T = [T; Tsim+(j-1)*Ts];
end
X = [];
for i = 1:Np
    X = [X; XYplot_ref(2*i-1,:)];
end
Y = [];
for i = 1:Np
    Y = [Y; XYplot_ref(2*i,:)];
end

X = [XYplot_sim(1,:); X];
Y = [XYplot_sim(2,:); Y];   
Vx0 = Velocity_sim*cos(Heading_sim);
Vy0 = Velocity_sim*sin(Heading_sim);
Yaw0 = Heading_sim;

[Velocity_updated, Heading_updated] = P2YV(0,0, T , X , Y , Vx0 , Vy0 , Yaw0, Np, 0, 0 );
end

== matlab function MPC_control/observer_of_plant/Subsystem_7/simulator_7/MPC_of_simulator_7/HQP ==
  data: r output; JE input; phi input; Fxh input; Qc input; U output; M input; Np input; Heading_updated input; Velocity_updated input; Rs input; Tsim input; select_MPC input; U_delay input
function [r,U] = HQP(JE ,phi,Fxh ,Qc ,M ,Np,Heading_updated ,Velocity_updated ,Rs ,Tsim, select_MPC, U_delay)
u1_max = 3*pi; u1_min = -3*pi;
u2_max =  1; u2_min = -1;
du1_inc = 3*pi;du1_dec = 3*pi;
du2_inc =  1;du2_dec =  1;
U_max = []; U_min = [];
for i = 1:Np
    U_max = [U_max; [u1_max; u2_max]];
    U_min = [U_min; [-u1_min; -u2_min]];
end

dU_plus = []; dU_minus = [];
for i = 1:Np
    dU_plus = [dU_plus; [U_delay(1) + du1_inc; U_delay(2) + du2_inc]];
    dU_minus = [dU_minus; [-U_delay(1) + du1_dec; -U_delay(2) + du2_dec;]];
end
N = [U_max;
      U_min;
      dU_plus;
      dU_minus;          
     ];
 
if Tsim > 0
    for i = 1: Np
        Rs(2*i-1,:) = Velocity_updated(i,:);
        Rs(2*i,:) = Heading_updated(i,:);
    end
end
% Rs(2,:) = Heading_updated;

JF = -2*phi'*Qc*(Rs-Fxh);
[u,lambda]= HQP(JE,JF,M,N);
U = u(1:2);
r = Rs(1:2,:);
end

== matlab function MPC_control/Passenger Vehicle/beta ==
  data: xdot input; beta output; ydot input; Velocity output
function [beta, Velocity]  = Velocity_Beta(xdot, ydot)
beta = 0; Velocity = 0;
Velocity = sqrt(xdot^2 + ydot^2);
xdot = abs(xdot);
beta = atan2(ydot, xdot);
end

== matlab function MPC_control/observer_of_plant/Subsystem_7/gate7 ==
  data: select_MPC input; state_MPC output; select_overlap input; state_overlap output; select_overlap2 input
function [state_MPC, state_overlap] = gate(select_MPC, select_overlap,select_overlap2)
model_num = 7;
if select_MPC == model_num
    state_MPC = 1;
else
    state_MPC = 0;
end

if select_overlap == model_num||select_overlap2 == model_num
    state_overlap = 1;
else
    state_overlap = 0;
end
end

== matlab function MPC_control/observer_of_plant/Subsystem_8/simulator_8/VH2P/YV2P ==
  data: Velocity input; LastVelocity input; Heading input; LastHeading input; Tsim input; LastTsim input; Lastpostion input; Position output
function Position  = YV2P(Velocity,LastVelocity, Heading, LastHeading, Tsim, LastTsim, Lastpostion)
if Tsim >= 0.1
    Position = zeros(2,1);
    X0 = Lastpostion(1,:); Y0 = Lastpostion(2,:);
    Vx0 = [LastVelocity*cos(LastHeading); Velocity*cos(Heading)];
    Vy0 = [LastVelocity*sin(LastHeading); Velocity*sin(Heading)];
    Yaw_sim = [LastHeading; Heading];
    T =[LastTsim; Tsim];
    [ X_tmp, Y_tmp] = YV2P( T, X0, Y0, Vx0, Vy0, Yaw_sim, zeros(2,1) );
    Position = [X_tmp(end,:); Y_tmp(end,:)];
else
    Position = [0; 0];
end
end

== matlab function MPC_control/observer_of_plant/Subsystem_8/simulator_8/YV_update/YV_update ==
  data: XYplot_ref input; Velocity_updated output; XYplot_sim input; Velocity_sim input; Heading_sim input; Ts input; Tsim input; Heading_updated output
function [Velocity_updated, Heading_updated] = VY_update(XYplot_ref, XYplot_sim, Velocity_sim, Heading_sim, Ts, Tsim)
Np = 6;
disp(sprintf('Simulation time : %2.1f sec',Tsim));
Heading_updated = zeros(Np,1); Velocity_updated = zeros(Np,1);
coder.extrinsic('P2YV');
T = [];

for j = 1:Np+1
    T = [T; Tsim+(j-1)*Ts];
end
X = [];
for i = 1:Np
    X = [X; XYplot_ref(2*i-1,:)];
end
Y = [];
for i = 1:Np
    Y = [Y; XYplot_ref(2*i,:)];
end

X = [XYplot_sim(1,:); X];
Y = [XYplot_sim(2,:); Y];   
Vx0 = Velocity_sim*cos(Heading_sim);
Vy0 = Velocity_sim*sin(Heading_sim);
Yaw0 = Heading_sim;

[Velocity_updated, Heading_updated] = P2YV(0,0, T , X , Y , Vx0 , Vy0 , Yaw0, Np, 0, 0 );
end

== matlab function MPC_control/observer_of_plant/Subsystem_8/simulator_8/MPC_of_simulator_8/HQP ==
  data: r output; JE input; phi input; Fxh input; Qc input; U output; M input; Np input; Heading_updated input; Velocity_updated input; Rs input; Tsim input; select_MPC input; U_delay input
function [r,U] = HQP(JE ,phi,Fxh ,Qc ,M ,Np,Heading_updated ,Velocity_updated ,Rs ,Tsim, select_MPC, U_delay)
u1_max = 3*pi; u1_min = -3*pi;
u2_max =  1; u2_min = -1;
du1_inc = 3*pi;du1_dec = 3*pi;
du2_inc =  1;du2_dec =  1;
U_max = []; U_min = [];
for i = 1:Np
    U_max = [U_max; [u1_max; u2_max]];
    U_min = [U_min; [-u1_min; -u2_min]];
end

dU_plus = []; dU_minus = [];
for i = 1:Np
    dU_plus = [dU_plus; [U_delay(1) + du1_inc; U_delay(2) + du2_inc]];
    dU_minus = [dU_minus; [-U_delay(1) + du1_dec; -U_delay(2) + du2_dec;]];
end
N = [U_max;
      U_min;
      dU_plus;
      dU_minus;          
     ];
 
if Tsim > 0
    for i = 1: Np
        Rs(2*i,:) = Heading_updated(i,:);
        Rs(2*i-1,:) = Velocity_updated(i,:);
    end
end
% Rs(2,:) = Heading_updated;

JF = -2*phi'*Qc*(Rs-Fxh);
[u,lambda]= HQP(JE,JF,M,N);
U = u(1:2);
r = Rs(1:2,:);
end
